simulink model "q2_JK"  (R2016b)
settings: Solver=VariableStepAuto  StartTime=0.0  StopTime=24  RelTol=1e-3
libraries: simulink_extras x4
settings Model: Creator=dell  LastModifiedBy=dell
settings OptimizationCC: BooleanDataType=off

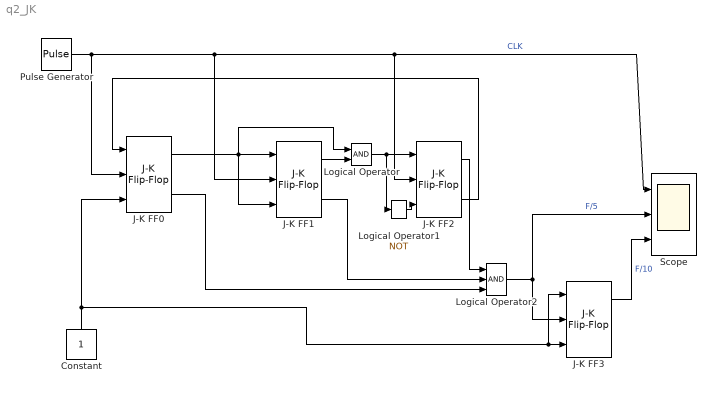
== system q2_JK ==
  Constant : Constant  OutDataTypeStr=boolean
  J-K FF{0..3} (4 alike) : simulink_extras/Flip Flops/J-K Flip-Flop  initial_condition=1
  Logical Operator : Logic  AllPortsSameDT=off  OutDataTypeStr=boolean
  Logical Operator1 : Logic  Operator=NOT  AllPortsSameDT=off  OutDataTypeStr=boolean
  Logical Operator2 : Logic  Inputs=3  AllPortsSameDT=off  OutDataTypeStr=boolean
  Pulse Generator : DiscretePulseGenerator
  Scope : Scope  NumInputPorts=3
  wires:
  J-K FF2/2 -> J-K FF0/1
  J-K FF1/1 -> Logical Operator/2
  J-K FF2/1 -> Logical Operator2/1
  J-K FF1/2 -> Logical Operator2/2
  J-K FF0/2 -> Logical Operator2/3
  Pulse Generator/1 -> J-K FF0/2, J-K FF1/2, Scope/1, J-K FF2/2  "CLK"
  Logical Operator/1 -> Logical Operator1/1, J-K FF2/1
  J-K FF0/1 -> Logical Operator/1, J-K FF1/3, J-K FF1/1
  Logical Operator1/1 -> J-K FF2/3
  Logical Operator2/1 -> Scope/2, J-K FF3/2  "F/5"
  Constant/1 -> J-K FF3/1, J-K FF3/3, J-K FF0/3
  J-K FF3/1 -> Scope/3  "F/10"
